simulink model "NLD2"  (R2022a)
settings: Solver=FixedStepDiscrete  StartTime=0.0  StopTime=xin.TimeInfo.End  RelTol=1e-3
values from neighbouring files (symbols this model uses):
  Ts = 1e-6    (= 1e-06)    [NLD1sim.m]    (also in NLD2sim.m; SPNF1sim.m; SPNF2sim.m)
undefined symbols (not defined in the file or in its folder): cols
libraries: simulink x12
settings Model: Creator=dileepan  LastModifiedBy=dileepan
settings SolverCC: AlgebraicLoopSolver=TrustRegion
settings DataIOCC: SaveFormat=Array  SaveOutput=off  SignalLogging=off  DSMLogging=off  SaveTime=off  ReturnWorkspaceOutputs=off
settings DebuggingCC: UnconnectedInputMsg=warning  UnconnectedOutputMsg=warning  UnconnectedLineMsg=warning  SFMachineParentedDataDiag=warning
settings RTWCC: DLArmComputeVersion=19.05

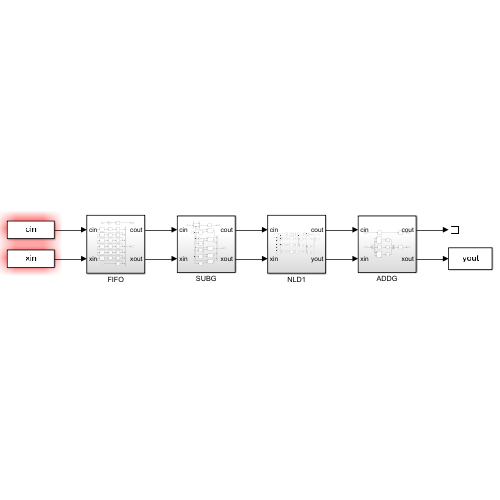
[thumbnail: Simulink's stored preview of the top-level diagram]
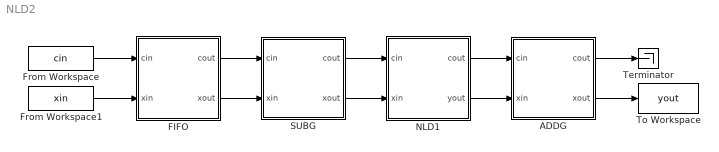
== system NLD2 ==
  ADDG : Subsystem
  FIFO : Subsystem
  From Workspace : FromWorkspace  VariableName=cin  SampleTime=Ts
  From Workspace1 : FromWorkspace  VariableName=xin  SampleTime=Ts
  NLD1 : Subsystem
  SUBG : Subsystem
  Terminator : Terminator
  To Workspace : ToWorkspace  VariableName=yout  SaveFormat=Timeseries  SampleTime=-1
  wires:
  FIFO/1(cout) -> SUBG/1(cin)
  FIFO/2(xout) -> SUBG/2(xin)
  SUBG/2(xout) -> NLD1/2(xin)
  SUBG/1(cout) -> NLD1/1(cin)
  From Workspace/1 -> FIFO/1(cin)
  From Workspace1/1 -> FIFO/2(xin)
  NLD1/1(cout) -> ADDG/1(cin)
  NLD1/2(yout) -> ADDG/2(xin)
  ADDG/2(xout) -> To Workspace/1
  ADDG/1(cout) -> Terminator/1

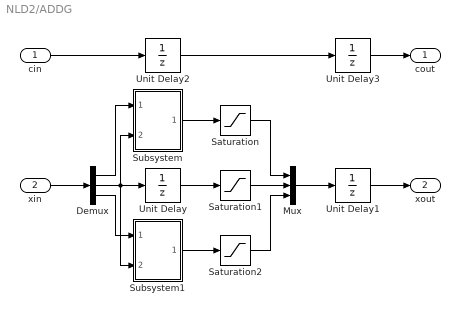
== system NLD2/ADDG ==
  cin : Inport
  xin : Inport  Port=2
  Demux : Demux  Outputs=3
  Mux : Mux  Inputs=3
  Saturation : Saturate  UpperLimit=intmax('uint8')  LowerLimit=intmin('uint8')  OutDataTypeStr=uint8
  Saturation1 : Saturate  UpperLimit=intmax('uint8')  LowerLimit=intmin('uint8')  OutDataTypeStr=uint8
  Saturation2 : Saturate  UpperLimit=intmax('uint8')  LowerLimit=intmin('uint8')  OutDataTypeStr=uint8
  Subsystem : Subsystem  TreatAsAtomicUnit=on  ReferencedSubsystem=add2
  Subsystem1 : Subsystem  TreatAsAtomicUnit=on  ReferencedSubsystem=add2
  Unit Delay{,1..3} (4 alike) : UnitDelay  SampleTime=-1  HasFrameUpgradeWarning=on
  cout : Outport
  xout : Outport  Port=2
  wires:
  xin/1 -> Demux/1
  Demux/2 -> Subsystem1/2, Subsystem/2, Unit Delay/1
  Demux/1 -> Subsystem/1
  Demux/3 -> Subsystem1/1
  Unit Delay1/1 -> xout/1
  cin/1 -> Unit Delay2/1
  Unit Delay2/1 -> Unit Delay3/1
  Unit Delay3/1 -> cout/1
  Subsystem/1 -> Saturation/1
  Subsystem1/1 -> Saturation2/1
  Unit Delay/1 -> Saturation1/1
  Saturation/1 -> Mux/1
  Saturation1/1 -> Mux/2
  Saturation2/1 -> Mux/3
  Mux/1 -> Unit Delay1/1

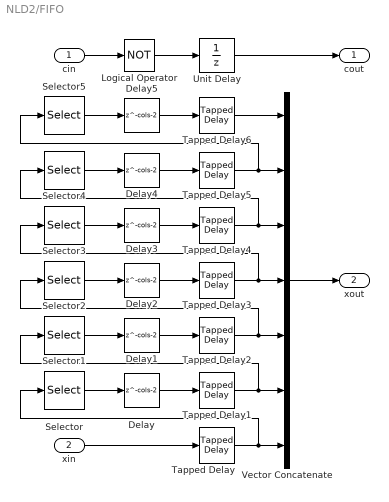
== system NLD2/FIFO ==
  cin : Inport
  xin : Inport  Port=2
  Delay{,1..5} (6 alike) : Delay  DelayLength=cols-2  UseCircularBuffer=on
  Logical Operator : Logic  Operator=NOT  IconShape=distinctive  AllPortsSameDT=off  OutDataTypeStr=boolean
  Selector{,1..5} (6 alike) : Selector  InputPortWidth=3  IndexOptions=Index vector (dialog)  Indices=1  OutputSizes=1
  Tapped Delay{,1..6} (7 alike) : simulink/Discrete/Tapped Delay  vinit=0.0  samptime=-1  NumDelays=2  DelayOrder=Oldest  includeCurrent=on
  Unit Delay : UnitDelay  SampleTime=-1  HasFrameUpgradeWarning=on
  Vector Concatenate : Concatenate  NumInputs=7  ConcatenateDimension=2
  cout : Outport
  xout : Outport  Port=2
  wires:
  Delay3/1 -> Tapped Delay4/1
  Selector1/1 -> Delay1/1
  Selector3/1 -> Delay3/1
  Tapped Delay6/1 -> Vector Concatenate/1
  Delay4/1 -> Tapped Delay5/1
  Selector/1 -> Delay/1
  Delay/1 -> Tapped Delay1/1
  Selector2/1 -> Delay2/1
  Selector5/1 -> Delay5/1
  Selector4/1 -> Delay4/1
  Delay2/1 -> Tapped Delay3/1
  Delay5/1 -> Tapped Delay6/1
  Delay1/1 -> Tapped Delay2/1
  xin/1 -> Tapped Delay/1
  Vector Concatenate/1 -> xout/1
  Unit Delay/1 -> cout/1
  Logical Operator/1 -> Unit Delay/1
  cin/1 -> Logical Operator/1
  Tapped Delay5/1 -> Vector Concatenate/2, Selector5/1
  Tapped Delay4/1 -> Vector Concatenate/3, Selector4/1
  Tapped Delay3/1 -> Vector Concatenate/4, Selector3/1
  Tapped Delay2/1 -> Vector Concatenate/5, Selector2/1
  Tapped Delay1/1 -> Vector Concatenate/6, Selector1/1
  Tapped Delay/1 -> Vector Concatenate/7, Selector/1

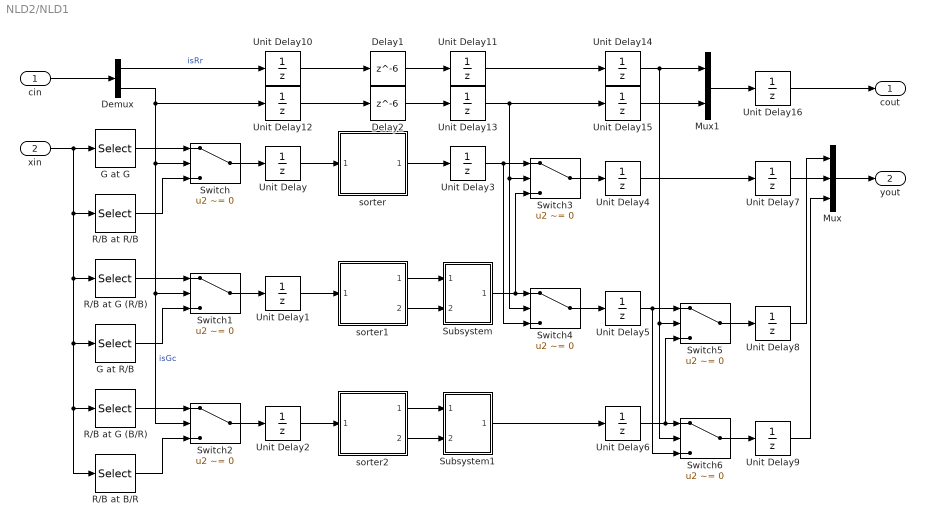
== system NLD2/NLD1 ==
  cin : Inport
  xin : Inport  Port=2
  Delay1 : Delay  DelayLength=6
  Delay2 : Delay  DelayLength=6
  Demux : Demux  Outputs=2
  G at G : Selector  InputPortWidth=25  IndexOptions=Index vector (dialog)  Indices=[7 9 13 13 13 17 19]  OutputSizes=1
  G at R/B : Selector  InputPortWidth=25  IndexOptions=Index vector (dialog)  Indices=[8 8 12 12 14 14 18 18]  OutputSizes=1
  Mux : Mux  Inputs=3
  Mux1 : Mux  Inputs=2
  R/B at B/R : Selector  InputPortWidth=25  IndexOptions=Index vector (dialog)  Indices=[7 7 9 9 17 17 19 19]  OutputSizes=1
  R/B at G (B/R) : Selector  InputPortWidth=25  IndexOptions=Index vector (dialog)  Indices=[6 8 8 10 16 18 18 20]  OutputSizes=1
  R/B at G (R/B) : Selector  InputPortWidth=25  IndexOptions=Index vector (dialog)  Indices=[2 4 12 12 14 14 22 24]  OutputSizes=1
  R/B at R/B : Selector  InputPortWidth=25  IndexOptions=Index vector (dialog)  Indices=[3 11 13 13 13 15 23]  OutputSizes=1
  Subsystem : Subsystem  TreatAsAtomicUnit=on  ReferencedSubsystem=mean2
  Subsystem1 : Subsystem  TreatAsAtomicUnit=on  ReferencedSubsystem=mean2
  Switch{,1..6} (7 alike) : Switch  Criteria=u2 ~= 0  SaturateOnIntegerOverflow=off  InputSameDT=off
  Unit Delay{,1..16} (17 alike) : UnitDelay  SampleTime=-1  HasFrameUpgradeWarning=on
  sorter : Subsystem  TreatAsAtomicUnit=on  ReferencedSubsystem=median7
  sorter1 : Subsystem  TreatAsAtomicUnit=on  ReferencedSubsystem=median8
  sorter2 : Subsystem  TreatAsAtomicUnit=on  ReferencedSubsystem=median8
  cout : Outport
  yout : Outport  Port=2
  wires:
  Switch3/1 -> Unit Delay4/1
  sorter1/1 -> Subsystem/1
  Delay1/1 -> Unit Delay11/1
  Unit Delay13/1 -> Unit Delay15/1, Switch3/2, Switch4/2
  G at G/1 -> Switch/1
  R/B at G (B/R)/1 -> Switch2/1
  Unit Delay14/1 -> Mux1/1, Switch5/2, Switch6/2
  Unit Delay7/1 -> Mux/2
  xin/1 -> G at G/1, R/B at R/B/1, R/B at G (R/B)/1, G at R/B/1, R/B at G (B/R)/1, R/B at B/R/1
  Unit Delay5/1 -> Switch6/3, Switch5/1
  G at R/B/1 -> Switch1/3
  Switch1/1 -> Unit Delay1/1
  Switch/1 -> Unit Delay/1
  Unit Delay2/1 -> sorter2/1
  R/B at R/B/1 -> Switch/3
  Unit Delay1/1 -> sorter1/1
  sorter2/2 -> Subsystem1/2
  Delay2/1 -> Unit Delay13/1
  Switch5/1 -> Unit Delay8/1
  Switch2/1 -> Unit Delay2/1
  Unit Delay10/1 -> Delay1/1
  Unit Delay4/1 -> Unit Delay7/1
  Unit Delay15/1 -> Mux1/2
  Switch6/1 -> Unit Delay9/1
  Demux/2 -> Switch/2, Switch1/2, Switch2/2, Unit Delay12/1  "isGc"
  sorter1/2 -> Subsystem/2
  Subsystem1/1 -> Unit Delay6/1
  sorter/1 -> Unit Delay3/1
  Unit Delay6/1 -> Switch5/3, Switch6/1
  Unit Delay3/1 -> Switch4/3, Switch3/1
  Unit Delay8/1 -> Mux/1
  Subsystem/1 -> Switch3/3, Switch4/1
  sorter2/1 -> Subsystem1/1
  Mux1/1 -> Unit Delay16/1
  Mux/1 -> yout/1
  R/B at B/R/1 -> Switch2/3
  Unit Delay12/1 -> Delay2/1
  Unit Delay9/1 -> Mux/3
  Switch4/1 -> Unit Delay5/1
  Demux/1 -> Unit Delay10/1  "isRr"
  Unit Delay11/1 -> Unit Delay14/1
  Unit Delay/1 -> sorter/1
  R/B at G (R/B)/1 -> Switch1/1
  Unit Delay16/1 -> cout/1
  cin/1 -> Demux/1

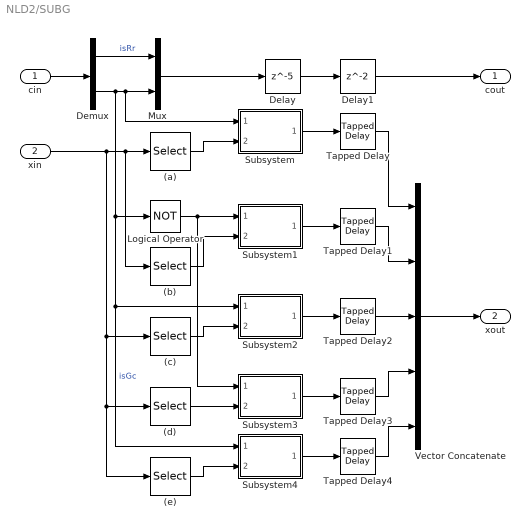
== system NLD2/SUBG ==
  cin : Inport
  xin : Inport  Port=2
  (a) : Selector  InputPortWidth=21  IndexOptions=Index vector (dialog)  Indices=[2 4:6 8]  OutputSizes=1
  (b) : Selector  InputPortWidth=21  IndexOptions=Index vector (dialog)  Indices=[5 7:9 11]  OutputSizes=1
  (c) : Selector  InputPortWidth=21  IndexOptions=Index vector (dialog)  Indices=[8 10:12 14]  OutputSizes=1
  (d) : Selector  InputPortWidth=21  IndexOptions=Index vector (dialog)  Indices=[11 13:15 17]  OutputSizes=1
  (e) : Selector  InputPortWidth=21  IndexOptions=Index vector (dialog)  Indices=[14 16:18 20]  OutputSizes=1
  Delay : Delay  DelayLength=5
  Delay1 : Delay
  Demux : Demux  Outputs=2
  Logical Operator : Logic  Operator=NOT  IconShape=distinctive  AllPortsSameDT=off  OutDataTypeStr=boolean
  Mux : Mux  Inputs=2
  Subsystem{,1..4} (5 alike) : Subsystem  ReferencedSubsystem=subG
  Tapped Delay{,1..4} (5 alike) : simulink/Discrete/Tapped Delay  vinit=0.0  samptime=-1  NumDelays=4  DelayOrder=Oldest  includeCurrent=on
  Vector Concatenate : Concatenate  NumInputs=5
  cout : Outport
  xout : Outport  Port=2
  wires:
  (d)/1 -> Subsystem3/2
  (c)/1 -> Subsystem2/2
  Demux/1 -> Mux/1  "isRr"
  Vector Concatenate/1 -> xout/1
  (b)/1 -> Subsystem1/2
  cin/1 -> Demux/1
  (e)/1 -> Subsystem4/2
  (a)/1 -> Subsystem/2
  Mux/1 -> Delay/1
  Subsystem/1 -> Tapped Delay/1
  Subsystem1/1 -> Tapped Delay1/1
  Subsystem2/1 -> Tapped Delay2/1
  Subsystem3/1 -> Tapped Delay3/1
  Tapped Delay2/1 -> Vector Concatenate/3
  Tapped Delay1/1 -> Vector Concatenate/2
  Tapped Delay4/1 -> Vector Concatenate/5
  Delay/1 -> Delay1/1
  Delay1/1 -> cout/1
  Tapped Delay/1 -> Vector Concatenate/1
  Tapped Delay3/1 -> Vector Concatenate/4
  Subsystem4/1 -> Tapped Delay4/1
  Logical Operator/1 -> Subsystem3/1, Subsystem1/1
  xin/1 -> (e)/1, (d)/1, (c)/1, (a)/1, (b)/1
  Demux/2 -> Subsystem4/1, Subsystem2/1, Logical Operator/1, Subsystem/1, Mux/2  "isGc"
